simulink model "Blinker_steuerung_1"  (R2015b)
settings: Solver=FixedStepAuto  StartTime=0.0  StopTime=inf  RelTol=1e-3
settings Model: Creator=guch0001  LastModifiedBy=scco1019

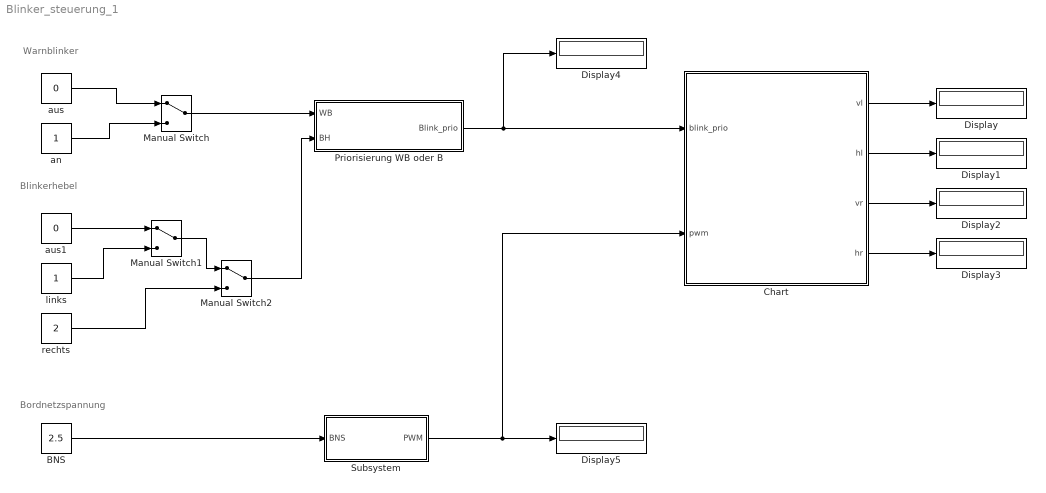
== system Blinker_steuerung_1 ==
  note: Bordnetzspannung
  note: Warnblinker
  note: Blinkerhebel
  BNS : Constant  Value=2.5
  Chart : Stateflow chart  TreatAsAtomicUnit=on
  Display{,1..5} (6 alike) : Display
  Manual Switch : ManualSwitch
  Manual Switch1 : ManualSwitch
  Manual Switch2 : ManualSwitch
  Priorisierung WB oder B : Subsystem
  Subsystem : Subsystem
  an : Constant
  aus : Constant  Value=0
  aus1 : Constant  Value=0
  links : Constant
  rechts : Constant  Value=2
  wires:
  aus/1 -> Manual Switch/1
  an/1 -> Manual Switch/2
  aus1/1 -> Manual Switch1/1
  links/1 -> Manual Switch1/2
  rechts/1 -> Manual Switch2/2
  Manual Switch1/1 -> Manual Switch2/1
  Manual Switch/1 -> Priorisierung WB oder B/1(WB)
  Manual Switch2/1 -> Priorisierung WB oder B/2(BH)
  Priorisierung WB oder B/1("Blink_prio ") -> Display4/1, Chart/1(blink_prio)
  Chart/4(hr) -> Display3/1
  Chart/1(vl) -> Display/1
  Chart/2(hl) -> Display1/1
  Chart/3(vr) -> Display2/1
  BNS/1 -> Subsystem/1(BNS)
  Subsystem/1(PWM) -> Chart/2(pwm), Display5/1

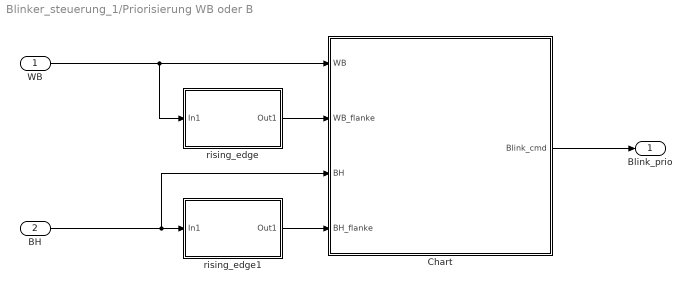
== system Blinker_steuerung_1/Priorisierung WB oder B ==
  WB : Inport
  BH : Inport  Port=2
  Chart : Stateflow chart  TreatAsAtomicUnit=on
  rising_edge : Subsystem
  rising_edge1 : Subsystem
  "Blink_prio " : Outport
  wires:
  BH/1 -> Chart/3(BH), rising_edge1/1(In1)
  WB/1 -> Chart/1(WB), rising_edge/1(In1)
  rising_edge/1(Out1) -> Chart/2(WB_flanke)
  rising_edge1/1(Out1) -> Chart/4(BH_flanke)
  Chart/1(Blink_cmd) -> "Blink_prio "/1

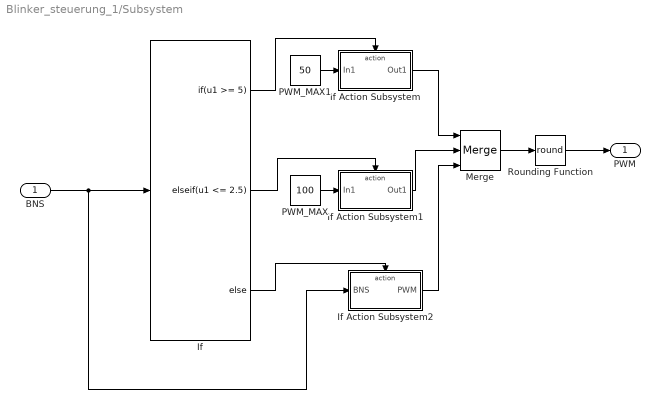
== system Blinker_steuerung_1/Subsystem ==
  BNS : Inport
  If : If  IfExpression=u1 >= 5  ElseIfExpressions=u1 <= 2.5
  If Action Subsystem : Subsystem  TreatAsAtomicUnit=on
  If Action Subsystem1 : Subsystem  TreatAsAtomicUnit=on
  If Action Subsystem2 : Subsystem  TreatAsAtomicUnit=on
  Merge : Merge  Inputs=3
  PWM_MAX : Constant  Value=100
  PWM_MAX1 : Constant  Value=50
  Rounding Function : Rounding  Operator=round
  PWM : Outport
  wires:
  BNS/1 -> If Action Subsystem2/1("BNS "), If/1
  If/1 -> If Action Subsystem/Action
  If Action Subsystem/1(Out1) -> Merge/1
  If/2 -> If Action Subsystem1/Action
  If Action Subsystem1/1(Out1) -> Merge/2
  If/3 -> If Action Subsystem2/Action
  If Action Subsystem2/1(PWM) -> Merge/3
  Merge/1 -> Rounding Function/1
  Rounding Function/1 -> PWM/1
  PWM_MAX/1 -> If Action Subsystem1/1(In1)
  PWM_MAX1/1 -> If Action Subsystem/1(In1)

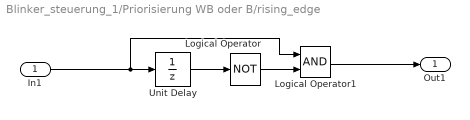
== system Blinker_steuerung_1/Priorisierung WB oder B/rising_edge ==
  In1 : Inport
  Logical Operator : Logic  Operator=NOT  AllPortsSameDT=off  OutDataTypeStr=boolean
  Logical Operator1 : Logic  AllPortsSameDT=off  OutDataTypeStr=boolean
  Unit Delay : UnitDelay  SampleTime=-1
  Out1 : Outport
  wires:
  In1/1 -> Logical Operator1/1, Unit Delay/1
  Unit Delay/1 -> Logical Operator/1
  Logical Operator/1 -> Logical Operator1/2
  Logical Operator1/1 -> Out1/1

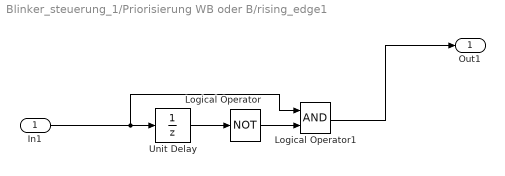
== system Blinker_steuerung_1/Priorisierung WB oder B/rising_edge1 ==
  In1 : Inport
  Logical Operator : Logic  Operator=NOT  AllPortsSameDT=off  OutDataTypeStr=boolean
  Logical Operator1 : Logic  AllPortsSameDT=off  OutDataTypeStr=boolean
  Unit Delay : UnitDelay  SampleTime=-1
  Out1 : Outport
  wires:
  Logical Operator1/1 -> Out1/1
  Logical Operator/1 -> Logical Operator1/2
  Unit Delay/1 -> Logical Operator/1
  In1/1 -> Unit Delay/1, Logical Operator1/1

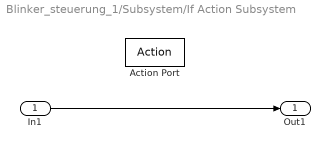
== system Blinker_steuerung_1/Subsystem/If Action Subsystem ==
  In1 : Inport
  Action Port : ActionPort  ActionType=then
  Out1 : Outport
  wires:
  In1/1 -> Out1/1

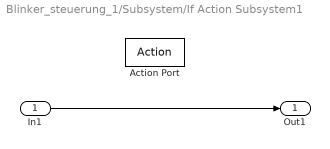
== system Blinker_steuerung_1/Subsystem/If Action Subsystem1 ==
  In1 : Inport
  Action Port : ActionPort  ActionType=elseif
  Out1 : Outport
  wires:
  In1/1 -> Out1/1

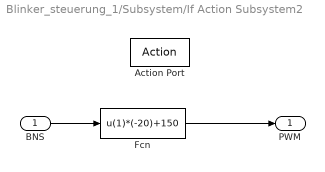
== system Blinker_steuerung_1/Subsystem/If Action Subsystem2 ==
  "BNS " : Inport
  Action Port : ActionPort  ActionType=else
  Fcn : Fcn  Expr=u(1)*(-20)+150
  PWM : Outport
  wires:
  "BNS "/1 -> Fcn/1
  Fcn/1 -> PWM/1

== stateflow chart Blinker_steuerung_1/Chart ==
  state state/
  (default) -> state
  (junction 4) -> state [order 2] : [blink_prio==1]
      | {vl=1;
      | hl=1;
      | vr=0;
      | hr=0;}
  (junction 4) -> state [order 1] : [blink_prio==0]
      | {vl=0;
      | hl=0;
      | vr=0;
      | hr=0;}
  (junction 4) -> state [order 3] : [blink_prio==3]
      | {vl=1;
      | hl=1;
      | vr=1;
      | hr=1;}
  (junction 4) -> state [order 4] : [blink_prio==2]
      | {vl=0;
      | hl=0;
      | vr=1;
      | hr=1;}
  state -> (junction 4)
  data: blink_prio input; vl output; hl output; vr output; hr output; pwm input

== stateflow chart Blinker_steuerung_1/Priorisierung WB oder B/Chart ==
  state RB_hat_Prio/
  state WB_hat_Prio/
  (default) -> RB_hat_Prio
  RB_hat_Prio -> (junction 16) [order 2]
  (junction 16) -> RB_hat_Prio [order 1] : [BH==1]{Blink_cmd=1;}
  (junction 16) -> RB_hat_Prio [order 2] : [BH==2]{Blink_cmd=2;}
  (junction 16) -> RB_hat_Prio [order 4] : {Blink_cmd=0;}
  (junction 16) -> RB_hat_Prio [order 3] : [WB==1]{Blink_cmd=3;}
  WB_hat_Prio -> RB_hat_Prio [order 1] : [BH_flanke==1]
  RB_hat_Prio -> WB_hat_Prio [order 1] : [WB_flanke==1]
  WB_hat_Prio -> (junction 4) [order 2]
  (junction 4) -> WB_hat_Prio [order 1] : [WB==1]{Blink_cmd=3;}
  (junction 4) -> WB_hat_Prio [order 4] : {Blink_cmd=0;}
  (junction 4) -> WB_hat_Prio [order 3] : [BH==2]{Blink_cmd=2;}
  (junction 4) -> WB_hat_Prio [order 2] : [BH==1]{Blink_cmd=1;}
  data: WB input; WB_flanke input; BH input; BH_flanke input; Blink_cmd output
